simulink model "BatteryHV_harness_model"  (R2023a)
settings: Solver=daessc  StartTime=0.0  StopTime=100*3600  RelTol=1e-3
PreLoadFcn:
  | BatteryHV_harness_setup
undefined symbols (not defined in the file): Minus, Plus
libraries: fl_lib x6, nesl_utility x5, simulink x2
settings Model: Creator=isaacito  LastModifiedBy=Jerikka
settings DataIOCC: DSMLogging=off
settings OptimizationCC: ReuseModelBlockBuffer=off
settings ModelReferenceCC: EnableRefExpFcnMdlSchedulingChecks=on
settings SimscapeCC: SimscapeLogType=all  SimscapeLogSimulationStatistics=on  SimscapeLogLimitData=off

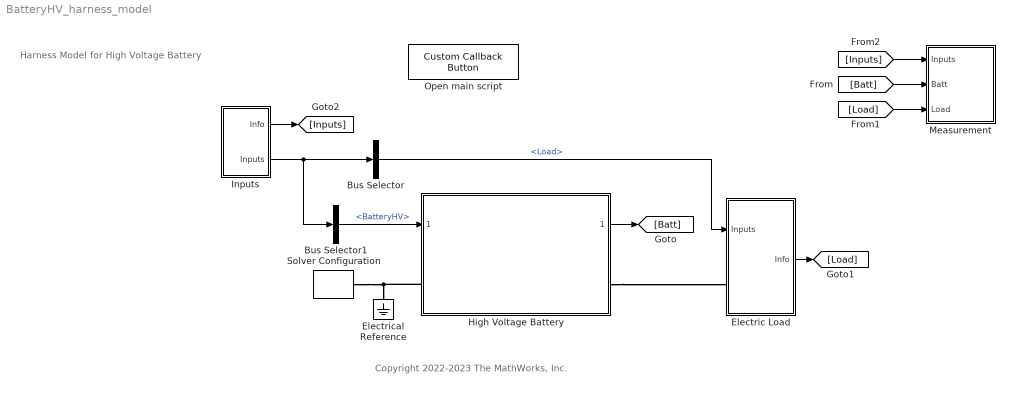
== system BatteryHV_harness_model ==
  note: Harness Model for High Voltage Battery
  note: Copyright 2022-2023 The MathWorks, Inc.
  Bus Selector : BusSelector  OutputSignals=Load
  Bus Selector1 : BusSelector  OutputSignals=BatteryHV
  Electric Load : Subsystem
  Electrical Reference : fl_lib/Electrical/Electrical Elements/Electrical Reference
  High Voltage Battery : Subsystem  ReferencedSubsystem=BatteryHV_refsub_System
      settings: OpenFcn=|
      | % Look under mask:
      | open_system(gcb, "force")
  Inputs : Subsystem
  Measurement : Subsystem
  Open main script : CustomCallbackButton  Configuration="{\"components\":[{\"name\":\"BackgroundImageComponent\",\"settings\":{\"image\":{\"size\":[0,0],\"src\":\"default\",\"srcOrientation\":\"Right\"},\"position\":[0,0,1,1]}},{\"name\":\"ButtonStateComponent\",\"settings\":{\"buttonType\":\"momentary\",\"clickFcn\":\"edit BatteryHV_main_script\\n\",\"onValue\":1,\"position\":[0,0,1,1],\"pressDelay\":\"500\",\"pressFcn\":\"\",\"repeatInterval\":\"0\",\"states\":[{\"horizontalAlignment\":\"center\",\"image\":{\"position\":[0,0,1,1],\"src\":\"default\",\"srcOrientation\":\"Right\"},\"label\":{\"color\":[0.01176470588,0.01176470588,0.01176470588,1],\"icon\":{\"size\":[0,0],\"src\":\"default\",\"srcOrientation\":\"Right\"},\"iconPlacement\":\"left\",\"text\":{\"content\":\"Main script\"}},\"labelOffset\":[0,0],\"verticalAlignment\":\"middle\"},{\"horizontalAlignment\":\"center\",\"image\":{\"position\":[0,0,1,1],\"src\":\"default\",\"srcOrientation\":\"Right\"},\"label\":{\"color\":[0.01176470588,0.01176470588,0.01176470588,1],\"icon\":{\"size\":[0,0],\"src\":\"default\",\"srcOrientation\":\"Right\"},\"iconPlacement\":\"left\",\"text\":{\"content\":\"Main script\"}},\"labelOffset\":[0,0],\"verticalAlignment\":\"middle\"},{\"horizontalAlignment\":\"center\",\"image\":{\"position\":[0,0,1,1],\"src\":\"default\",\"srcOrientation\":\"Right\"},\"label\":{\"color\":[0.01176470588,0.01176470588,0.01176470588,1],\"icon\":{\"size\":[0,0],\"src\":\"default\",\"srcOrientation\":\"Right\"},\"iconPlacement\":\"left\",\"text\":{\"content\":\"Main script\"}},\"labelOffset\":[0,0],\"verticalAlignment\":\"middle\"},{\"horizontalAlignment\":\"center\",\"image\":{\"position\":[0,0,1,1],\"src\":\"default\",\"srcOrientation\":\"Right\"},\"label\":{\"color\":[0.01176470588,0.01176470588,0.01176470588,1],\"icon\":{\"size\":[0,0],\"src\":\"default\",\"srcOrientation\":\"Right\"},\"iconPlacement\":\"left\",\"text\":{\"content\":\"Main script\"}},\"labelOffset\":[0,0],\"verticalAlignment\":\"middle\"}]}},{\"name\":\"ForegroundImageComponent\",\"settings\":{\"image\":{\"size\":[0,0],\"src\":\"default\",\"srcOrientation\":\"Right\"},\"isForeground\":1,\"position\":[0,0,1,1]}}],\"settings\":{\"BindingType\":\"standalone\",\"backgroundColor\":[244,244,244,1],\"backgroundOffset\":0.2,\"backgroundOpacity\":1,\"fixedAspectRatio\":\"off\",\"foregroundColor\":[0.01176470588,0.01176470588,0.01176470588,1],\"migratedFromLegacy\":true,\"useBackgroundColor\":true,\"variant\":\"callback\",\"version\":\"R2023a\"},\"type\":\"Button\"}"  CustomBackgroundColor="{\"color\":[0.9568627451,0.9568627451,0.9568627451],\"show\":true}"
  Solver Configuration : nesl_utility/Solver Configuration  PhysicalDomain=network_engine_domain  SubClassName=solver  LeftPortType=input  RightPortType=generic  Tones=[]  Harmonics=[]  SimulateNoise=off  Profile=off  UseLocalSampling=off  EnableSwitchedLinearOptims=on  FrequencyDomain=off  UseCCode=off  RelTol=0.001  AbsTol=0.001  MinStep=1e-09  ToWorkspace=off  RevertToSquareIcSolve=off  NumHomotopyIterations=100  PhasorMode=off  PhasorModeNumHarmonics=1  ConsistencySolver=NEWTON_FTOL  IndexReductionMethod=DerivativeReplacement  DoDC=off  ResidualTolerance=1e-09  ConsistencyTolSource=GLOBAL  ConsistencyAbsTol=0.001  ConsistencyRelTol=0.001  ConsistencyTolFactor=0.001  UseLocalSolver=off  LocalSolverChoice=NE_BACKWARD_EULER_ADVANCER  ResolveIndetEquations=on  FunctionEvalNumThread=1  LocalSolverSampleTime=0.001  DoFixedCost=off  MaxNonlinIter=3  MaxModeIter=2  ComputeImpulses=off  ImpulseIterations=2  LinearAlgebra=auto  LinearAlgebraNumThread=0  EquationFormulation=NE_TIME_EF  DelaysMemoryBudget=1024  AutomaticFiltering=on  FilteringTimeConstant=0.001  PartitionStorageMethod=AS_NEEDED  PartitionMemoryBudget=1024  PartitionMethod=ROBUST
      settings: AttributesFormatString=Local solver: %<UseLocalSolver>
  wires:
  High Voltage Battery/1 -> [Batt]
  [Batt] -> Measurement/2(Batt)
  Electric Load/1(Info) -> [Load]
  [Load] -> Measurement/3(Load)
  [Inputs] -> Measurement/1(Inputs)
  Inputs/1(Info) -> [Inputs]
  Inputs/2(Inputs) -> Bus Selector/1, Bus Selector1/1
  Bus Selector/1 -> Electric Load/1(Inputs)  "<Load>"
  Bus Selector1/1 -> High Voltage Battery/1  "<BatteryHV>"
  connections:
  High Voltage Battery/LConn1 -- Electrical Reference/LConn1 -- Solver Configuration/RConn1
  High Voltage Battery/RConn1 -- Electric Load/LConn1

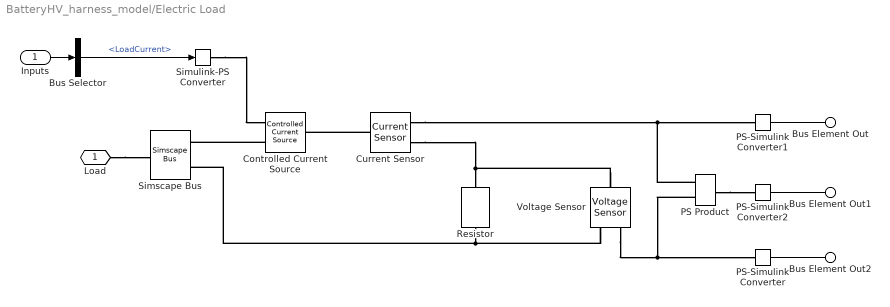
== system BatteryHV_harness_model/Electric Load ==
  Inputs : Inport
  Bus Selector : BusSelector  OutputSignals=LoadCurrent
  Controlled Current Source : fl_lib/Electrical/Electrical Sources/Controlled Current Source
  Current Sensor : fl_lib/Electrical/Electrical Sensors/Current Sensor
  PS Product : fl_lib/Physical Signals/Functions/PS Product
  PS-Simulink Converter : nesl_utility/PS-Simulink Converter  PhysicalDomain=network_engine_domain  SubClassName=ps_output  LeftPortType=input  RightPortType=output  PseudoPeriodic=off  Frequencies=[]  VectorFormat=inherit  Unit=V  AffineConversion=off
  PS-Simulink Converter1 : nesl_utility/PS-Simulink Converter  PhysicalDomain=network_engine_domain  SubClassName=ps_output  LeftPortType=input  RightPortType=output  PseudoPeriodic=off  Frequencies=[]  VectorFormat=inherit  Unit=A  AffineConversion=off
  PS-Simulink Converter2 : nesl_utility/PS-Simulink Converter  PhysicalDomain=network_engine_domain  SubClassName=ps_output  LeftPortType=input  RightPortType=output  PseudoPeriodic=off  Frequencies=[]  VectorFormat=inherit  Unit=kW  AffineConversion=off
  Resistor : fl_lib/Electrical/Electrical Elements/Resistor  R=1 Ohm  i_specify=off  i_priority=None  i=0 A  i_nominal_specify=off  i_nominal_unit=A  i_nominal_value=1  v_specify=off  v_priority=None  v=0 V  v_nominal_specify=off  v_nominal_unit=V  v_nominal_value=1
  Simscape Bus : SimscapeBus  HierarchyStrings=Plus;Minus  ConnectionType=Bus: Bus_HighVoltage
  Simulink-PS Converter : nesl_utility/Simulink-PS Converter  PhysicalDomain=network_engine_domain  SubClassName=ps_input  LeftPortType=input  RightPortType=output  PseudoPeriodic=off  Frequencies=[]  NoiseDistribution=none  NoiseParameters=[]  Unit=A  AffineConversion=off  FilteringAndDerivatives=provide  SimscapeFilterOrder=1  InputFilterTimeConstant=0.001  UdotUserProvided=0
  Voltage Sensor : fl_lib/Electrical/Electrical Sensors/Voltage Sensor
  Load : PMIOPort  Side=Left
  Bus Element Out : Outport  PortName=Info  Element=Curr
  Bus Element Out1 : Outport  PortName=Info  Element=Pwr
  Bus Element Out2 : Outport  PortName=Info  Element=V
  wires:
  PS-Simulink Converter1/1 -> Bus Element Out/1
  PS-Simulink Converter2/1 -> Bus Element Out1/1
  PS-Simulink Converter/1 -> Bus Element Out2/1
  Inputs/1 -> Bus Selector/1
  Bus Selector/1 -> Simulink-PS Converter/1  "<LoadCurrent>"
  connections:
  Load/RConn1 -- Simscape Bus/RConn1
  Controlled Current Source/RConn2 -- Simscape Bus/LConn1
  Resistor/RConn1 -- Voltage Sensor/RConn2 -- Simscape Bus/LConn2
  Simulink-PS Converter/RConn1 -- Controlled Current Source/RConn1
  Current Sensor/LConn1 -- Controlled Current Source/LConn1
  Current Sensor/RConn2 -- Voltage Sensor/LConn1 -- Resistor/LConn1
  Voltage Sensor/RConn1 -- PS Product/LConn2 -- PS-Simulink Converter/LConn1
  Current Sensor/RConn1 -- PS Product/LConn1 -- PS-Simulink Converter1/LConn1
  PS Product/RConn1 -- PS-Simulink Converter2/LConn1

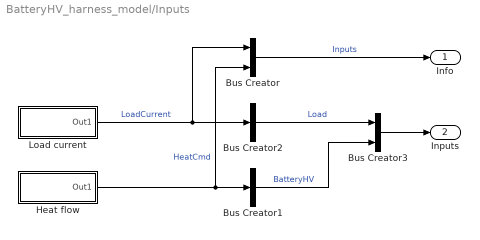
== system BatteryHV_harness_model/Inputs ==
  Bus Creator : BusCreator  Inputs=2
  Bus Creator1 : BusCreator  Inputs=1
  Bus Creator2 : BusCreator  Inputs=1
  Bus Creator3 : BusCreator  Inputs=2
  Heat flow : Subsystem  mask(Continuous Multi-Step Signal){dataPoints=[0 1 -1], deltaT=1}
      mask prompts: dataPoints "Data points"; deltaT "Interpolation step [s]"
      mask help:
      | This block generates a signal consisting of smoothly connected flat segments. Data points parameter takes an N-by-3 matrix where each row specifies a flat segment. First column and second column define start and end time of the segment, respectively. Third column defines the value of the segment. Second column can also be NaN to define a point value. Flat segments and point values are smoothly interpolated by Akima spline with the specified interpolation step.
      |
      | For example, a matrix [0 1 5; 3 nan 9; 6 8 7] for Data points defines a signal as follows. First row defines a flat segment from t=0 to t=1 of value 5. Second row defines a point at t=3 of value 9. Third row defines a flat segment from t=6 to t=8 of value 7.
      mask init:
      | sig = SignalDesigner("ContinuousMultiStep");
      | 
      | % Initialization function can access parameter names directly
      | sig.XYData = dataPoints;
      | sig.DeltaX = deltaT;
      | 
      | update(sig)
      | 
      | SignalSourceBlockCallback.setDataToLookupTableBlock( ...
      |   SignalObject = sig, ...
      |   PathToBlock = [gcb '/1-D Lookup Table']);
      mask DialogControl Control3 Prompt: horizontal spacer 1
      mask DialogControl Control4 Prompt: horizontal spacer 2
      mask DialogControl Control5 Prompt: horizontal spacer 3
      mask DialogControl PlotButton Prompt: Plot
      mask DialogControl PlotButton Callback: SignalSourceBlockCallback.plotContinuousMultiStep(gcb);
      mask Display: disp("Continuous" + newline + "Multi-Step")
  Load current : Subsystem  mask(Continuous Multi-Step Signal){dataPoints=[0 3600 -17.6470588235294], deltaT=0.2}
      mask prompts: dataPoints "Data points"; deltaT "Interpolation step [s]"
      mask help:
      | This block generates a signal consisting of smoothly connected flat segments. Data points parameter takes an N-by-3 matrix where each row specifies a flat segment. First column and second column define start and end time of the segment, respectively. Third column defines the value of the segment. Second column can also be NaN to define a point value. Flat segments and point values are smoothly interpolated by Akima spline with the specified interpolation step.
      |
      | For example, a matrix [0 1 5; 3 nan 9; 6 8 7] for Data points defines a signal as follows. First row defines a flat segment from t=0 to t=1 of value 5. Second row defines a point at t=3 of value 9. Third row defines a flat segment from t=6 to t=8 of value 7.
      mask init: same as BatteryHV_harness_model/Inputs/Heat flow
      mask DialogControl Control3 Prompt: horizontal spacer 1
      mask DialogControl Control4 Prompt: horizontal spacer 2
      mask DialogControl Control5 Prompt: horizontal spacer 3
      mask DialogControl PlotButton Prompt: Plot
      mask DialogControl PlotButton Callback: SignalSourceBlockCallback.plotContinuousMultiStep(gcb);
      mask Display: disp("Continuous" + newline + "Multi-Step")
  Info : Outport
  Inputs : Outport  Port=2
  wires:
  Load current/1(Out1) -> Bus Creator2/1, Bus Creator/1  "LoadCurrent"
  Heat flow/1(Out1) -> Bus Creator1/1, Bus Creator/2  "HeatCmd"
  Bus Creator/1 -> Info/1  "Inputs"
  Bus Creator2/1 -> Bus Creator3/1  "Load"
  Bus Creator1/1 -> Bus Creator3/2  "BatteryHV"
  Bus Creator3/1 -> Inputs/1

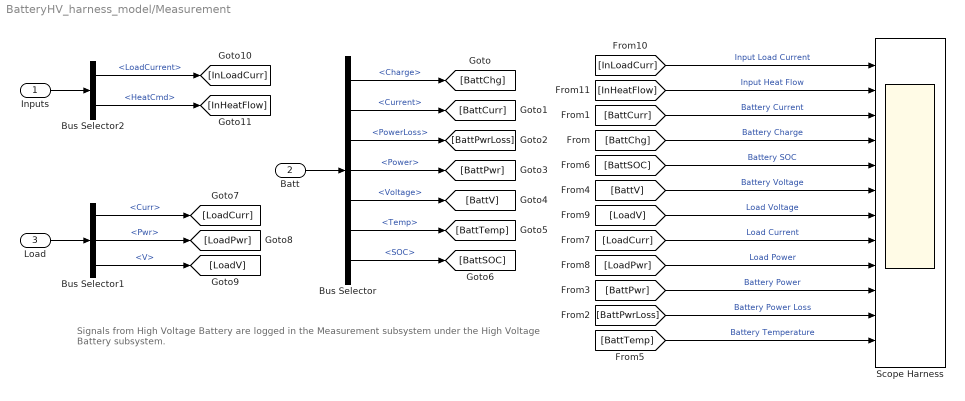
== system BatteryHV_harness_model/Measurement ==
  note: Signals from High Voltage Battery are logged in
      | the Measurement subsystem under the High Voltage Battery subsystem.
  Inputs : Inport
  Batt : Inport  Port=2
  Load : Inport  Port=3
  Bus Selector : BusSelector  OutputSignals=Charge,Current,PowerLoss,Power,Voltage,Temp,SOC
  Bus Selector1 : BusSelector  OutputSignals=Curr,Pwr,V
  Bus Selector2 : BusSelector  OutputSignals=LoadCurrent,HeatCmd
  Scope Harness : Scope  NumInputPorts=12
  wires:
  Batt/1 -> Bus Selector/1
  Bus Selector/1 -> [BattChg]  "<Charge>"
  Bus Selector/2 -> [BattCurr]  "<Current>"
  Bus Selector/3 -> [BattPwrLoss]  "<PowerLoss>"
  Bus Selector/4 -> [BattPwr]  "<Power>"
  Bus Selector/5 -> [BattV]  "<Voltage>"
  Bus Selector/6 -> [BattTemp]  "<Temp>"
  Bus Selector/7 -> [BattSOC]  "<SOC>"
  Load/1 -> Bus Selector1/1
  Bus Selector1/1 -> [LoadCurr]  "<Curr>"
  Bus Selector1/2 -> [LoadPwr]  "<Pwr>"
  Bus Selector1/3 -> [LoadV]  "<V>"
  [BattCurr] -> Scope Harness/3  "Battery Current"
  [BattChg] -> Scope Harness/4  "Battery Charge"
  [BattSOC] -> Scope Harness/5  "Battery SOC"
  [BattV] -> Scope Harness/6  "Battery Voltage"
  [LoadV] -> Scope Harness/7  "Load Voltage"
  [LoadCurr] -> Scope Harness/8  "Load Current"
  [LoadPwr] -> Scope Harness/9  "Load Power"
  [BattPwr] -> Scope Harness/10  "Battery Power"
  [BattPwrLoss] -> Scope Harness/11  "Battery Power Loss"
  [BattTemp] -> Scope Harness/12  "Battery Temperature"
  Inputs/1 -> Bus Selector2/1
  Bus Selector2/1 -> [InLoadCurr]  "<LoadCurrent>"
  [InLoadCurr] -> Scope Harness/1  "Input Load Current"
  Bus Selector2/2 -> [InHeatFlow]  "<HeatCmd>"
  [InHeatFlow] -> Scope Harness/2  "Input Heat Flow"

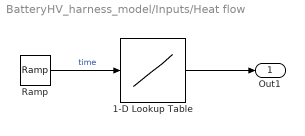
== system BatteryHV_harness_model/Inputs/Heat flow ==
  1-D Lookup Table : Lookup_n-D  NumberOfTableDimensions=1  BreakpointsForDimension1="[0  1]"  Table=[-1 -1]  InternalRulePriority=Speed  RndMeth=Simplest
  Ramp : simulink/Sources/Ramp  slope=1  start=0  InitialOutput=0
      settings: AttributesFormatString=|
      | Slope: %<slope>
      | Start time: %<start>
      | Initial output: %<InitialOutput>
  Out1 : Outport
  wires:
  Ramp/1 -> 1-D Lookup Table/1  "time"
  1-D Lookup Table/1 -> Out1/1

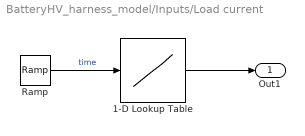
== system BatteryHV_harness_model/Inputs/Load current ==
  1-D Lookup Table : Lookup_n-D  NumberOfTableDimensions=1  BreakpointsForDimension1="[0  3600]"  Table="[-17.6471     -17.6471]"  InternalRulePriority=Speed  RndMeth=Simplest
  Ramp : simulink/Sources/Ramp  slope=1  start=0  InitialOutput=0
      settings: AttributesFormatString=|
      | Slope: %<slope>
      | Start time: %<start>
      | Initial output: %<InitialOutput>
  Out1 : Outport
  wires:
  Ramp/1 -> 1-D Lookup Table/1  "time"
  1-D Lookup Table/1 -> Out1/1
